simulink subsystem "Sensors_ThorneFleissner"  (R2020b)
settings: Solver=VariableStepAuto  StartTime=0.0  StopTime=10.0  RelTol=1e-3
settings Model: Creator=rthom  LastModifiedBy=rthom

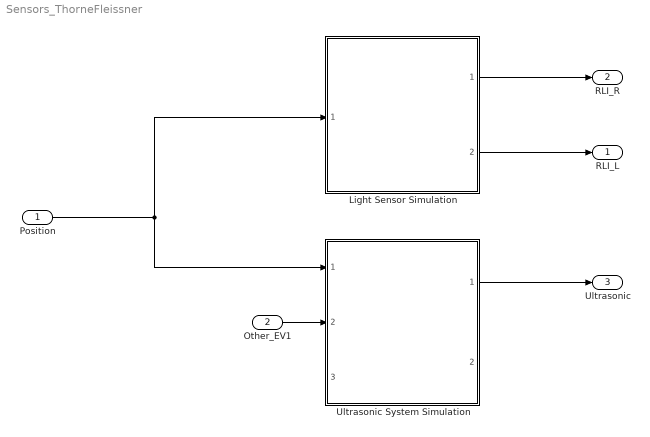
== system Sensors_ThorneFleissner ==
  Position : Inport
  Other_EV1 : Inport  Port=2
  Light Sensor Simulation : Subsystem  ReferencedSubsystem=Light_Sensor_Simulation_ThorneFleissner
  Ultrasonic System Simulation : Subsystem  ReferencedSubsystem=Ultrasonic_System_Simulation_ThorneFleissner
  RLI_L : Outport
  RLI_R : Outport  Port=2
  Ultrasonic : Outport  Port=3
  wires:
  Ultrasonic System Simulation/1 -> Ultrasonic/1
  Position/1 -> Ultrasonic System Simulation/1, Light Sensor Simulation/1
  Light Sensor Simulation/1 -> RLI_R/1
  Light Sensor Simulation/2 -> RLI_L/1
  Other_EV1/1 -> Ultrasonic System Simulation/2
